simulink library "threeTetherGroundStation_cl"  (R2018b)
settings: Solver=VariableStepAuto  StartTime=0.0  StopTime=10.0  RelTol=1e-3
libraries: vrlib x3, eulAng2RotMat_ul x1, massSpringDamper_ul x1
settings Model: Creator=mcobb  LastModifiedBy=mcobb

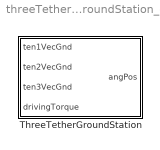
== system threeTetherGroundStation_cl ==
  ThreeTetherGroundStation : Subsystem  mask{r1=[1 0 0], r2=[0 1 0], r3=[0 -1 0], J=100, b=0, theta0=0, omega0=0}
      mask prompts: r1 "Tether 1 attach position vec"; r2 "Tether 2 attach position vec"; r3 "Tether 3 attach position vec"; J "Rotational Inertia"; b "Rotational Damping Coefficient"; theta0 "Initial position [rad]"; omega0 "Initial velocity [rad/s]"
      mask DialogControl Container3 Prompt: Tether Attachment Points

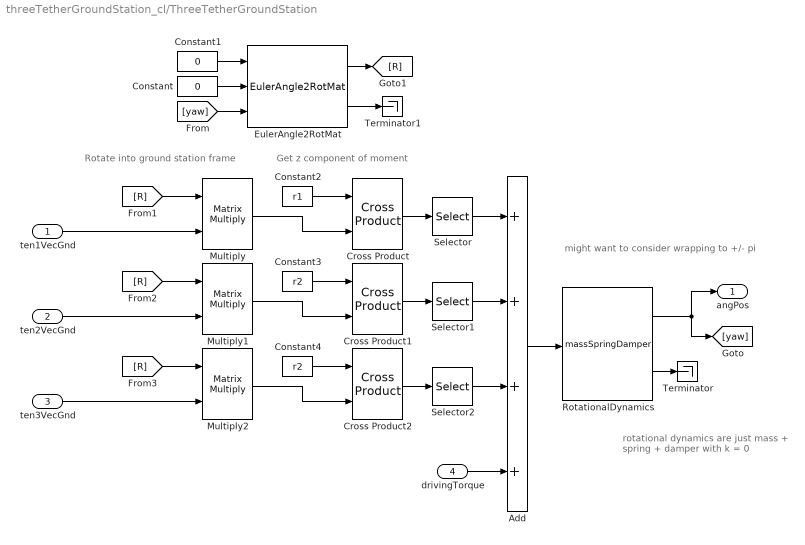
== system threeTetherGroundStation_cl/ThreeTetherGroundStation ==
  note: Get z component of moment
  note: Rotate into ground station frame
  note: rotational dynamics are just
      | mass + spring + damper with k = 0
  note: might want to consider wrapping to +/- pi
  ten1VecGnd : Inport
  ten2VecGnd : Inport  Port=2
  ten3VecGnd : Inport  Port=3
  drivingTorque : Inport  Port=4
  Add : Sum  Inputs=++++
  Constant : Constant  Value=0
  Constant1 : Constant  Value=0
  Constant2 : Constant  Value=r1
  Constant3 : Constant  Value=r2
  Constant4 : Constant  Value=r2
  Cross Product : vrlib/Utilities/Cross Product
      settings: SourceProductBaseCode=VR
  Cross Product1 : vrlib/Utilities/Cross Product
      settings: SourceProductBaseCode=VR
  Cross Product2 : vrlib/Utilities/Cross Product
      settings: SourceProductBaseCode=VR
  EulerAngle2RotMat : eulAng2RotMat_ul/EulerAngle2RotMat  SystemSampleTime=-1
  Multiply : Product  Multiplication=Matrix(*)
  Multiply1 : Product  Multiplication=Matrix(*)
  Multiply2 : Product  Multiplication=Matrix(*)
  RotationalDynamics : massSpringDamper_ul/massSpringDamper  m=J  b=b  k=0  x0=theta0  xDot0=omega0
  Selector : Selector  InputPortWidth=3  IndexOptions=Index vector (dialog)  Indices=3  OutputSizes=1
  Selector1 : Selector  InputPortWidth=3  IndexOptions=Index vector (dialog)  Indices=3  OutputSizes=1
  Selector2 : Selector  InputPortWidth=3  IndexOptions=Index vector (dialog)  Indices=3  OutputSizes=1
  Terminator : Terminator
  Terminator1 : Terminator
  angPos : Outport
  wires:
  ten1VecGnd/1 -> Multiply/2
  ten2VecGnd/1 -> Multiply1/2
  ten3VecGnd/1 -> Multiply2/2
  Selector1/1 -> Add/2
  Selector/1 -> Add/1
  Selector2/1 -> Add/3
  Add/1 -> RotationalDynamics/1
  RotationalDynamics/2 -> Terminator/1
  RotationalDynamics/1 -> [yaw], angPos/1
  drivingTorque/1 -> Add/4
  [yaw] -> EulerAngle2RotMat/3
  Constant/1 -> EulerAngle2RotMat/2
  Constant1/1 -> EulerAngle2RotMat/1
  EulerAngle2RotMat/2 -> Terminator1/1
  EulerAngle2RotMat/1 -> [R]
  [R] -> Multiply/1
  Multiply/1 -> Cross Product/2
  [R] -> Multiply1/1
  [R] -> Multiply2/1
  Multiply2/1 -> Cross Product2/2
  Multiply1/1 -> Cross Product1/2
  Cross Product/1 -> Selector/1
  Constant2/1 -> Cross Product/1
  Cross Product2/1 -> Selector2/1
  Cross Product1/1 -> Selector1/1
  Constant3/1 -> Cross Product1/1
  Constant4/1 -> Cross Product2/1
